simulink model "Controller"  (R2024b)
settings: Solver=ode45  StartTime=0.0  StopTime=25  RelTol=1e-3
undefined symbols (not defined in the file): drv, gbox, kd, ki, kp, mld, mot, rads2rpm, sens, step_gain, tl, Ts
settings Model: Creator=andre  LastModifiedBy=andre

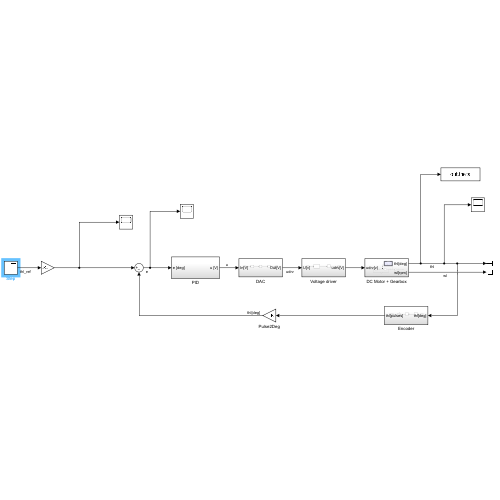
[thumbnail: Simulink's stored preview of the top-level diagram]
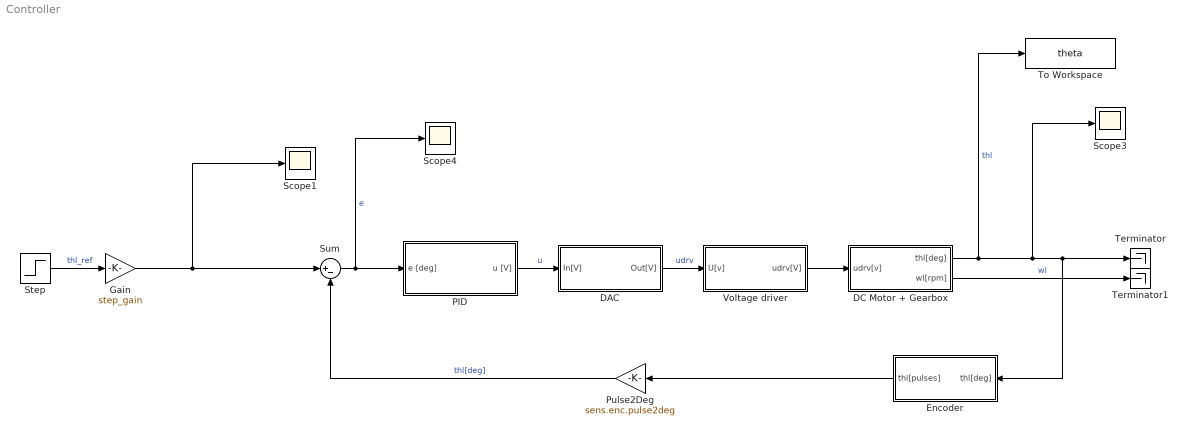
== system Controller ==
  DAC : Subsystem
  DC Motor + Gearbox : Subsystem
  Encoder : Subsystem
  Gain : Gain  Gain=step_gain
  PID : Subsystem
  Pulse2Deg : Gain  Gain=sens.enc.pulse2deg
  Scope1 : Scope
  Scope3 : Scope
  Scope4 : Scope
  Step : Step  Time=0  SampleTime=0
  Sum : Sum  Inputs=|+-
  Terminator : Terminator
  Terminator1 : Terminator
  To Workspace : ToWorkspace  VariableName=theta  SaveFormat=Timeseries  SampleTime=Ts
  Voltage driver : Subsystem
  wires:
  Step/1 -> Gain/1  "thl_ref"
  Sum/1 -> Scope4/1, PID/1(e [deg])  "e"
  PID/1(u [V]) -> DAC/1(In[V])  "u"
  DAC/1(Out[V]) -> Voltage driver/1(U[v])  "udrv"
  Voltage driver/1(udrv[V]) -> DC Motor + Gearbox/1(udrv[v])
  DC Motor + Gearbox/1(thl[deg]) -> To Workspace/1, Scope3/1, Terminator/1, Encoder/1(thl[deg])  "thl"
  DC Motor + Gearbox/2(wl[rpm]) -> Terminator1/1  "wl"
  Gain/1 -> Scope1/1, Sum/1
  Encoder/1(thl[pulses]) -> Pulse2Deg/1
  Pulse2Deg/1 -> Sum/2  "thl[deg]"

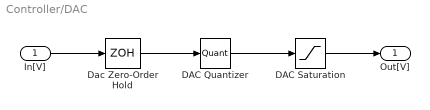
== system Controller/DAC ==
  In[V] : Inport
  DAC Quantizer : Quantizer  QuantizationInterval=20/(2^16-1)
  DAC Saturation : Saturate  UpperLimit=10  LowerLimit=-10
  Dac Zero-Order Hold : ZeroOrderHold  SampleTime=Ts
  Out[V] : Outport
  wires:
  In[V]/1 -> Dac Zero-Order Hold/1
  DAC Saturation/1 -> Out[V]/1
  DAC Quantizer/1 -> DAC Saturation/1
  Dac Zero-Order Hold/1 -> DAC Quantizer/1

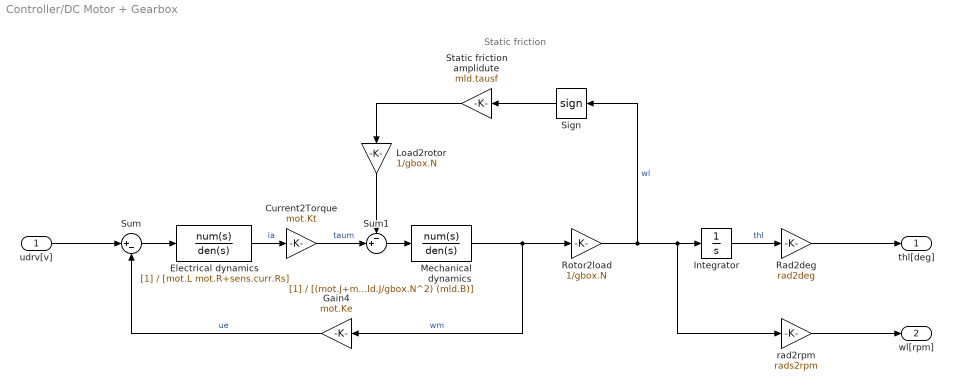
== system Controller/DC Motor + Gearbox ==
  note: Static friction
  udrv[v] : Inport
  " Sign" : Signum  ZeroCross=off
  Current2Torque : Gain  Gain=mot.Kt
  Electrical dynamics : TransferFcn  Denominator=[mot.L mot.R+sens.curr.Rs]
  Gain4 : Gain  Gain=mot.Ke
  Integrator : Integrator
  Load2rotor : Gain  Gain=1/gbox.N
  Mechanical dynamics : TransferFcn  Denominator=[(mot.J+mld.J/gbox.N^2) (mld.B)]
  Rad2deg : Gain  Gain=rad2deg
  Rotor2load : Gain  Gain=1/gbox.N
  Static friction amplidute : Gain  Gain=mld.tausf
  Sum : Sum  Inputs=|+-
  Sum1 : Sum  Inputs=-+|
  rad2rpm : Gain  Gain=rads2rpm
  thl[deg] : Outport
  wl[rpm] : Outport  Port=2
  wires:
  udrv[v]/1 -> Sum/1
  Sum/1 -> Electrical dynamics/1
  Electrical dynamics/1 -> Current2Torque/1  "ia"
  Current2Torque/1 -> Sum1/2  "taum"
  Load2rotor/1 -> Sum1/1
  " Sign"/1 -> Static friction amplidute/1
  Static friction amplidute/1 -> Load2rotor/1
  Sum1/1 -> Mechanical dynamics/1
  Mechanical dynamics/1 -> Gain4/1, Rotor2load/1  "wm"
  Gain4/1 -> Sum/2  "ue"
  Rad2deg/1 -> thl[deg]/1
  rad2rpm/1 -> wl[rpm]/1
  Integrator/1 -> Rad2deg/1  "thl"
  Rotor2load/1 -> " Sign"/1, rad2rpm/1, Integrator/1  "wl"

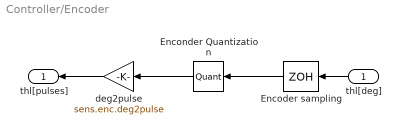
== system Controller/Encoder ==
  thl[deg] : Inport
  Encoder sampling : ZeroOrderHold  SampleTime=Ts
  Enconder Quantization : Quantizer  QuantizationInterval=sens.enc.pulse2deg
  deg2pulse : Gain  Gain=sens.enc.deg2pulse
  thl[pulses] : Outport
  wires:
  thl[deg]/1 -> Encoder sampling/1
  Enconder Quantization/1 -> deg2pulse/1
  deg2pulse/1 -> thl[pulses]/1
  Encoder sampling/1 -> Enconder Quantization/1

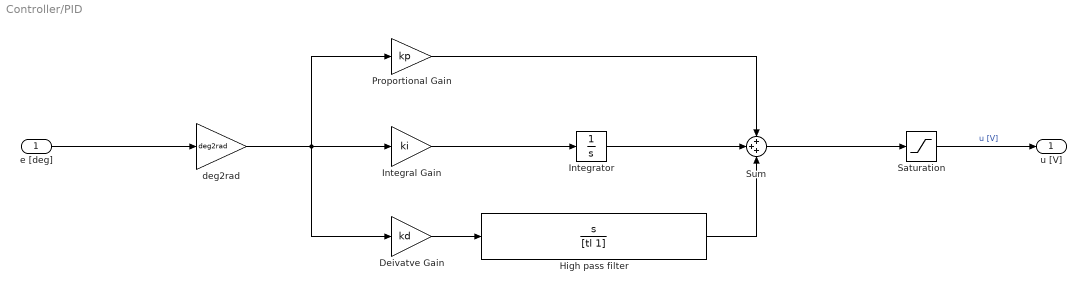
== system Controller/PID ==
  e [deg] : Inport
  Deivatve Gain : Gain  Gain=kd
  High pass filter : TransferFcn  Numerator=[1 0]  Denominator=[tl 1]
  Integral Gain : Gain  Gain=ki
  Integrator : Integrator
  Proportional Gain : Gain  Gain=kp
  Saturation : Saturate  UpperLimit=10  LowerLimit=-10
  Sum : Sum  Inputs=+++
  deg2rad : Gain  Gain=deg2rad
  u [V] : Outport
  wires:
  Deivatve Gain/1 -> High pass filter/1
  e [deg]/1 -> deg2rad/1
  Integrator/1 -> Sum/2
  Saturation/1 -> u [V]/1  "u [V]"
  deg2rad/1 -> Deivatve Gain/1, Proportional Gain/1, Integral Gain/1
  High pass filter/1 -> Sum/3
  Integral Gain/1 -> Integrator/1
  Proportional Gain/1 -> Sum/1
  Sum/1 -> Saturation/1

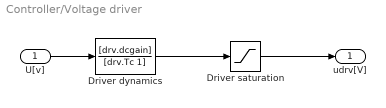
== system Controller/Voltage driver ==
  U[v] : Inport
  Driver dynamics : TransferFcn  Numerator=[drv.dcgain]  Denominator=[drv.Tc 1]
  Driver saturation : Saturate  UpperLimit=12  LowerLimit=-12
  udrv[V] : Outport
  wires:
  U[v]/1 -> Driver dynamics/1
  Driver dynamics/1 -> Driver saturation/1
  Driver saturation/1 -> udrv[V]/1
